simulink model "configuracionFeedbackV2"  (R2021b)
settings: Solver=ode45  StartTime=0.0  StopTime=10  RelTol=1e-3
PreLoadFcn:
  | f_tono = 500;
  | Fs = 44100;
InitFcn:
  | f_tono = 500;
  | Fs = 44100;
undefined symbols (not defined in the file or in its folder): SzEstimado
settings Model: Creator=Alejo  LastModifiedBy=ValeOieni

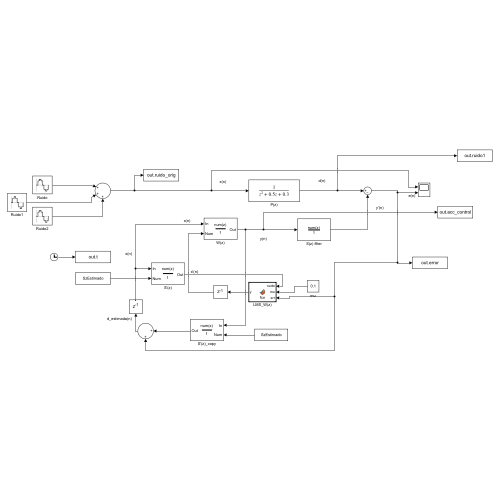
[thumbnail: Simulink's stored preview of the top-level diagram]
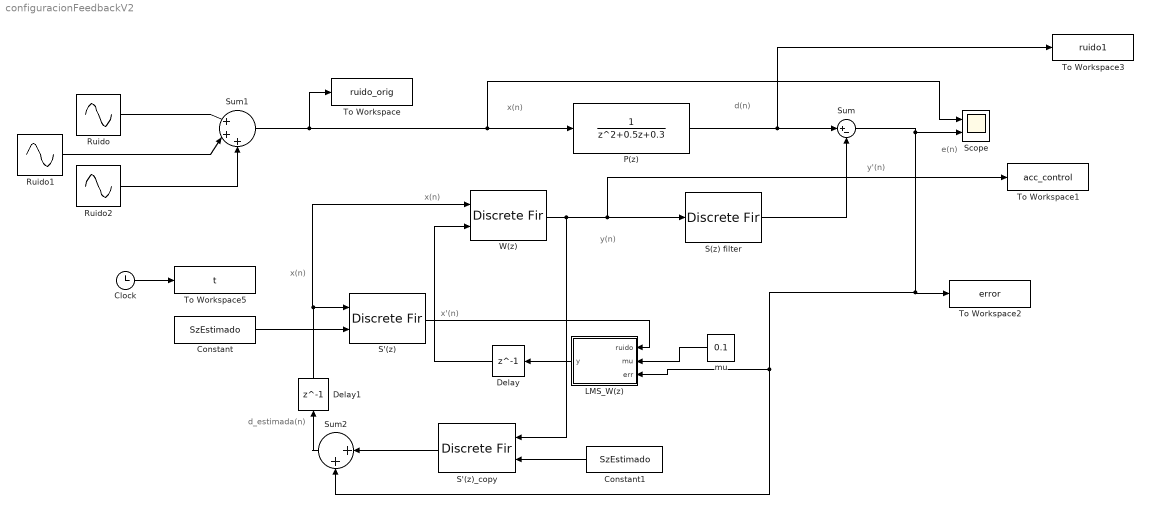
== system configuracionFeedbackV2 ==
  note: d_estimada(n)
  note: e(n)
  note: x'(n)
  note: x(n)
  note: y(n)
  note: y'(n)
  note: x(n)
  note: d(n)
  note: x(n)
  Clock : Clock
  Constant : Constant  Value=SzEstimado  SampleTime=1/Fs
  Constant1 : Constant  Value=SzEstimado  SampleTime=1/Fs
  Delay : Delay  DelayLength=1  InitialCondition=0
  Delay1 : Delay  DelayLength=1  InitialCondition=0
  LMS_W(z) : MATLAB Function  TreatAsAtomicUnit=on
  P(z) : DiscreteTransferFcn  Denominator="[1 0.5  0.3]"
  Ruido : Sin  Frequency=f_tono*(2*pi)  SampleTime=1/Fs
  Ruido1 : Sin  Frequency=2*f_tono*(2*pi)  SampleTime=1/Fs
  Ruido2 : Sin  Amplitude=2  Frequency=0.3*f_tono*(2*pi)  SampleTime=1/Fs
  S'(z) : DiscreteFir  CoefSource=Input port  SampleTime=1/Fs
      settings: InputPortMap=u0,u1
  S'(z)_copy : DiscreteFir  CoefSource=Input port  SampleTime=1/Fs
      settings: InputPortMap=u0,u1
  S(z) filter : DiscreteFir  Coefficients=[0 0 -.5 .5 -.3 .2 -.1 .5 -.5]  InputProcessing=Columns as channels (frame based)  SampleTime=1/Fs
  Scope : Scope  NumInputPorts=2
  Sum : Sum  Inputs=|+-
  Sum1 : Sum  Inputs=|+++
  Sum2 : Sum  Inputs=|++
  To Workspace : ToWorkspace  VariableName=ruido_orig  SampleTime=-1
      settings: Save2DSignal=2-D array (concatenate along first dimension)
  To Workspace1 : ToWorkspace  VariableName=acc_control  SampleTime=-1
      settings: Save2DSignal=2-D array (concatenate along first dimension)
  To Workspace2 : ToWorkspace  VariableName=error  SampleTime=-1
      settings: Save2DSignal=2-D array (concatenate along first dimension)
  To Workspace3 : ToWorkspace  VariableName=ruido1  SampleTime=-1
      settings: Save2DSignal=2-D array (concatenate along first dimension)
  To Workspace5 : ToWorkspace  VariableName=t  SampleTime=-1
      settings: Save2DSignal=2-D array (concatenate along first dimension)
  W(z) : DiscreteFir  CoefSource=Input port  SampleTime=1/Fs
      settings: InputPortMap=u0,u1
  mu : Constant  Value=0.1  SampleTime=1/Fs
  wires:
  S'(z)/1 -> LMS_W(z)/1(ruido)
  Ruido2/1 -> Sum1/3
  Ruido1/1 -> Sum1/2
  Constant/1 -> S'(z)/2
  Ruido/1 -> Sum1/1
  Sum/1 -> LMS_W(z)/3(err), Sum2/2, To Workspace2/1, Scope/2
  S(z) filter/1 -> Sum/2
  Constant1/1 -> S'(z)_copy/2
  Sum2/1 -> Delay1/1
  Sum1/1 -> To Workspace/1, P(z)/1, Scope/1
  LMS_W(z)/1(y) -> Delay/1
  W(z)/1 -> S'(z)_copy/1, S(z) filter/1, To Workspace1/1
  Clock/1 -> To Workspace5/1
  Delay/1 -> W(z)/2
  S'(z)_copy/1 -> Sum2/1
  Delay1/1 -> W(z)/1, S'(z)/1
  mu/1 -> LMS_W(z)/2(mu)
  P(z)/1 -> To Workspace3/1, Sum/1

== matlab function configuracionFeedbackV2/LMS_W(z) ==
  data: ruido input; mu input; y output; err input
function y = fcn(ruido, mu, err)
    L = 32;
    %Pesos w_n
    persistent w_n
    if isempty(w_n)
        w_n = zeros(1, L); % inicializa w en cero, largo L
    end
    %Vector de ruido
    persistent x
    if isempty(x)
        x = zeros(1, L); % inicializa x en cero, largo L
    end
    %Vaciado de x
    x(2:L) = x(1:L-1);
    x(1) = ruido;
    %Actualizacion
    xvar = x;
    w = w_n;
    w = w + mu*err*xvar;   
    w_n = w;
    %Asignación a la salida
    y = w;
end
